simulink model "plant_block_2024"  (R2024b)
settings: Solver=ode1  StartTime=0.0  StopTime=3000  RelTol=1e-3  EnableMultiTasking=on
libraries: slpidlib x3
settings Model: SimulationMode=external  Creator=Dro  LastModifiedBy=s4580656
settings SolverCC: AlgebraicLoopSolver=TrustRegion
settings DataIOCC: LimitDataPoints=on  SaveFormat=Array  SignalLoggingSaveFormat=ModelDataLogs  ReturnWorkspaceOutputs=off  SignalLoggingName=sigsOut
settings OptimizationCC: ExpressionDepthLimit=2147483647  InitFltsAndDblsToZero=on
settings DebuggingCC: SaveWithParameterizedLinksMsg=none  UnderspecifiedInitializationDetection=Classic  MergeDetectMultiDrivingBlocksExec=none  SignalResolutionControl=TryResolveAllWithWarning  MultiTaskDSMMsg=warning  MultiTaskCondExecSysMsg=none  FcnCallInpInsideContextMsg=warning  UnconnectedInputMsg=warning  UnconnectedOutputMsg=warning  UnconnectedLineMsg=warning  StateNameClashWarn=warning  SFUnexpectedBacktrackingDiag=warning  SFNoUnconditionalDefaultTransitionDiag=warning  SFExecutionAtInitializationDiag=none  ArithmeticOperatorsInVariantConditions=warning
settings HardwareCC: ProdBitPerLong=64  ProdHWDeviceType=Intel->x86-64 (Linux 64)  TargetBitPerLong=64  TargetBitPerPointer=64  TargetIntDivRoundTo=Zero  TargetEndianess=LittleEndian  TargetWordSize=64  TargetHWDeviceType=Intel->x86-64
settings ModelReferenceCC: EnableRefExpFcnMdlSchedulingChecks=on  PropagateSignalLabelsOutOfModel=off
settings SFSimCC: SimUseLocalCustomCode=off  CustomCodeUndefinedFunction=UseInterfaceOnly
settings RTWCC: Description=Simulink Desktop Real-Time  SystemTargetFile=sldrt.tlc  TemplateMakefile=sldrt.tmf  RTWUseLocalCustomCode=off  RTWCompilerOptimization=on  GPUComputeCapability=3.5
settings CodeAppCC: MaxIdLength=95  StateflowObjectComments=on
settings SimulinkDesktopRealTimeCC: TargetLibSuffix=_sldrt.a  TargetPreCompLibLocation=C:\Program Files\MATLAB\R2024b\toolbox\sldrt\lib\win64  TargetLangStandard=C89/C90 (ANSI)  ModelReferenceCompliant=off  ParMdlRefBuildCompliant=on  CompOptLevelCompliant=off  SupportVariableSizeSignals=off
settings ConfigComp: CovMetricSettings=dw  CovSaveCumulativeToWorkspaceVar=on  CovSaveSingleToWorkspaceVar=on  CovExternalEMLEnable=off

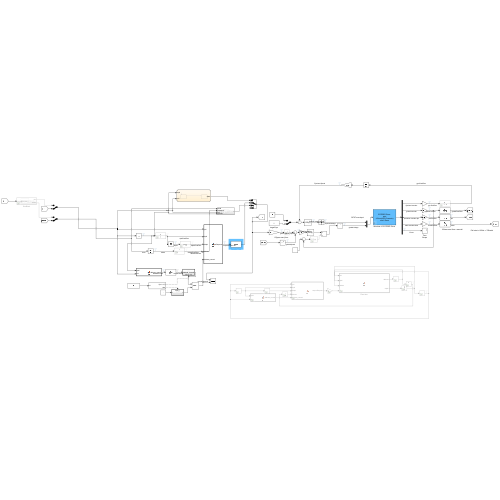
[thumbnail: Simulink's stored preview of the top-level diagram]
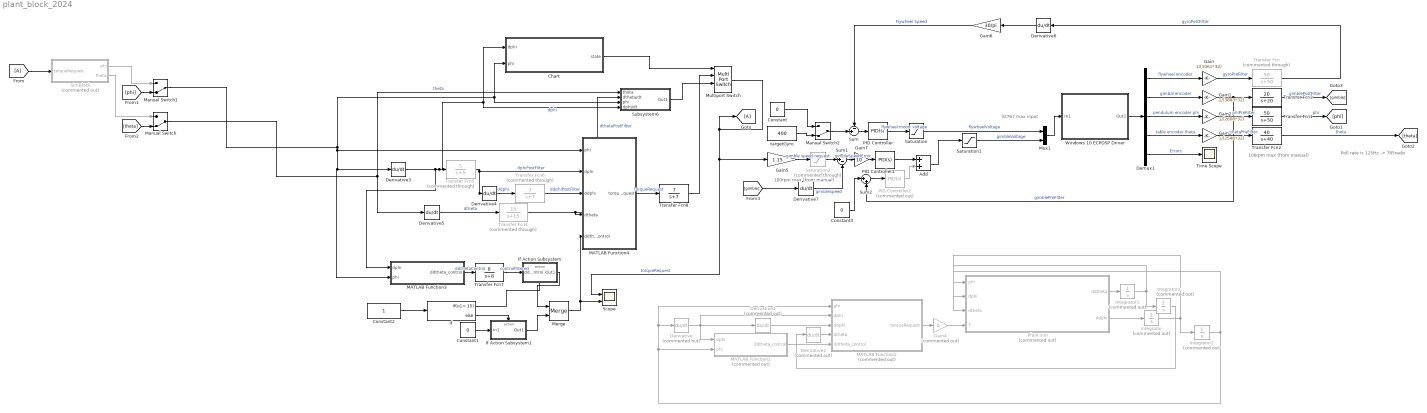
== system plant_block_2024 ==
  note: 100rpm max (from manual)
  note: 32767 max input
  note: Poll rate is 125Hz -> 785rad/s
  note: 100rpm max (from manual)
  Add : Sum
  Chart : Stateflow chart  TreatAsAtomicUnit=on
  Constant : Constant  Value=0
  Constant1 : Constant  Value=0
  Constant2 : Constant
  Constant3 : Constant  Value=0
  Demux1 : Demux  Outputs=5
      settings: DisplayOption=none
  Derivative : Derivative  Commented=on
  Derivative1 : Derivative  Commented=on
  Derivative2 : Derivative  Commented=on
  Derivative{3..7} (5 alike) : Derivative
  From : From
  Gain : Gain  Gain=1/(1061*32)
  Gain1 : Gain  Gain=1/(3883*32)
  Gain2 : Gain  Gain=1/(2608*32)
  Gain3 : Gain  Gain=1/(2546*32)
  Gain4 : Gain  Commented=on  Gain=0
  Gain5 : Gain  Gain=1.15
  Gain6 : Gain  Gain=30/pi
  Gain7 : Gain  Gain=10
  Goto : Goto
  If : If  IfExpression=u1< 15
  If Action Subsystem : Subsystem  TreatAsAtomicUnit=on
  If Action Subsystem1 : Subsystem  TreatAsAtomicUnit=on
  Integrator : Integrator  Commented=on
  Integrator1 : Integrator  Commented=on
  Integrator2 : Integrator  Commented=on  InitialCondition=pi
  Integrator3 : Integrator  Commented=on
  MATLAB Function1 : MATLAB Function  Commented=on  TreatAsAtomicUnit=on
  MATLAB Function2 : MATLAB Function  Commented=on  TreatAsAtomicUnit=on
  MATLAB Function3 : MATLAB Function  TreatAsAtomicUnit=on
  MATLAB Function4 : MATLAB Function  TreatAsAtomicUnit=on
  Manual Switch : ManualSwitch  CurrentSetting=0
  Manual Switch1 : ManualSwitch  CurrentSetting=0
  Manual Switch2 : ManualSwitch  CurrentSetting=0
  Merge : Merge  InitialOutput=[1]
  Multiport Switch : MultiPortSwitch  SaturateOnIntegerOverflow=off  InputSameDT=off
  Mux1 : Mux  Inputs=2
  PID Controller : slpidlib/PID Controller  Controller=PID  Form=Parallel  TimeDomain=Continuous-time  UseExternalTs=off  SampleTime=-1  IntegratorMethod=Forward Euler  FilterMethod=Forward Euler  ControllerParametersSource=internal  P=5500  I=100  UseKiTs=off  D=1  UseExternalDerivativeSource=off  N=100  UseFilter=on  TunerSelectOption=Transfer Function Based (PID Tuner App)  InitialConditionSource=internal  InitialConditionForIntegrator=0  InitialConditionForFilter=0  DifferentiatorICPrevScaledInput=0  ExternalReset=none  TrackingMode=off  Kt=1  LimitOutput=off  SatLimitsSource=internal  UpperSaturationLimit=32000  LowerSaturationLimit=-32000  LinearizeAsGain=on  AntiWindupMode=none  Kb=1  LimitIntegrator=off  UpperIntegratorSaturationLimit=inf  LowerIntegratorSaturationLimit=-inf  POutMin=[]  POutMax=[]  IOutMin=[]  IOutMax=[]  DOutMin=[]  DOutMax=[]  NOutMin=[]  NOutMax=[]  SumOutMin=[]  SumOutMax=[]  SaturationOutMin=[]  SaturationOutMax=[]  PParamMin=[]  PParamMax=[]  IParamMin=[]  IParamMax=[]  DParamMin=[]  DParamMax=[]  NParamMin=[]  NParamMax=[]  KbParamMin=[]  KbParamMax=[]  KtParamMin=[]  KtParamMax=[]  KbOutMin=[]  KbOutMax=[]  KtOutMin=[]  KtOutMax=[]  IntegratorOutMin=[]  IntegratorOutMax=[]  FilterOutMin=[]  FilterOutMax=[]  SumI1OutMin=[]  SumI1OutMax=[]  SumI2OutMin=[]  SumI2OutMax=[]  SumI3OutMin=[]  SumI3OutMax=[]  SumI4OutMin=[]  SumI4OutMax=[]  SumDOutMin=[]  SumDOutMax=[]  DifferentiatorOutMin=[]  DifferentiatorOutMax=[]  FilterDiffOutCoefMin=[]  FilterDiffOutCoefMax=[]  ReciprocalOutMin=[]  ReciprocalOutMax=[]  SumDenOutMin=[]  SumDenOutMax=[]  SumNumOutMin=[]  SumNumOutMax=[]  DivideOutMin=[]  DivideOutMax=[]  UdiffTsProdOutMin=[]  UdiffTsProdOutMax=[]  NTsProdOutMin=[]  NTsProdOutMax=[]  UintegralTsProdOutMin=[]  UintegralTsProdOutMax=[]  UngainTsProdOutMin=[]  UngainTsProdOutMax=[]  ClampingZeroOutDataTypeStr=Inherit: Inherit via back propagation  ClampingZeroOutMin=[]  ClampingZeroOutMax=[]  FilterDenConstantOutDataTypeStr=Inherit: Inherit via back propagation  FilterDenConstantOutMin=[]  FilterDenConstantOutMax=[]  PCopyOutDataTypeStr=Inherit: Inherit via back propagation  PCopyOutMin=[]  PCopyOutMax=[]  NCopyOutDataTypeStr=Inherit: Inherit via back propagation  NCopyOutMin=[]  NCopyOutMax=[]  IntegratorContinuousStateAttributes=''  IntegratorStateMustResolveToSignalObject=off  IntegratorRTWStateStorageClass=Auto  FilterContinuousStateAttributes=''  FilterStateMustResolveToSignalObject=off  FilterRTWStateStorageClass=Auto  ParallelPVariant=InternalParameters  IdealPVariant=Disabled  IVariant=InternalParameters  DVariant=InternalParameters  IntegratorVariant=Continuous  SatVariant=Disabled  AWVariant=Passthrough  PCopyVariant=Disabled  TRVariant=Disabled  FdbkBlocksVariant=Forward  IdealPFdbkVariant=Disabled  SatFdbkVariant=Disabled  DerivativeFilterVariant=ContFilter  NVariant=InternalParameters  NCopyVariant=Disabled  FilterICVariant=InternalICsFilter  IntegratorICVariant=InternalICs  ExternalResetVariant=Disabled  TRSumVariant=Passthrough  SumFdbkVariant=Disabled  SumVariant=Sum_PID  TsampFilterVariant=InternalTs  TsampNgainVariant=Passthrough  TsampIntegralVariant=Disabled_SignalSpec  ExternalSaturationOutDataTypeStr=Inherit: Same as second input  DerivativeSourceVariant=ErrorSignal  PreIntVariant=InternalPreInt
  PID Controller1 : slpidlib/PID Controller  Controller=PID  Form=Parallel  TimeDomain=Continuous-time  UseExternalTs=off  SampleTime=-1  IntegratorMethod=Forward Euler  FilterMethod=Forward Euler  ControllerParametersSource=internal  P=2500  I=50  UseKiTs=off  D=0  UseExternalDerivativeSource=off  N=100  UseFilter=on  TunerSelectOption=Transfer Function Based (PID Tuner App)  InitialConditionSource=internal  InitialConditionForIntegrator=0  InitialConditionForFilter=0  DifferentiatorICPrevScaledInput=0  ExternalReset=none  TrackingMode=off  Kt=1  LimitOutput=off  SatLimitsSource=internal  UpperSaturationLimit=23500  LowerSaturationLimit=-23500  LinearizeAsGain=on  AntiWindupMode=none  Kb=1  LimitIntegrator=off  UpperIntegratorSaturationLimit=inf  LowerIntegratorSaturationLimit=-inf  POutMin=[]  POutMax=[]  IOutMin=[]  IOutMax=[]  DOutMin=[]  DOutMax=[]  NOutMin=[]  NOutMax=[]  SumOutMin=[]  SumOutMax=[]  SaturationOutMin=[]  SaturationOutMax=[]  PParamMin=[]  PParamMax=[]  IParamMin=[]  IParamMax=[]  DParamMin=[]  DParamMax=[]  NParamMin=[]  NParamMax=[]  KbParamMin=[]  KbParamMax=[]  KtParamMin=[]  KtParamMax=[]  KbOutMin=[]  KbOutMax=[]  KtOutMin=[]  KtOutMax=[]  IntegratorOutMin=[]  IntegratorOutMax=[]  FilterOutMin=[]  FilterOutMax=[]  SumI1OutMin=[]  SumI1OutMax=[]  SumI2OutMin=[]  SumI2OutMax=[]  SumI3OutMin=[]  SumI3OutMax=[]  SumI4OutMin=[]  SumI4OutMax=[]  SumDOutMin=[]  SumDOutMax=[]  DifferentiatorOutMin=[]  DifferentiatorOutMax=[]  FilterDiffOutCoefMin=[]  FilterDiffOutCoefMax=[]  ReciprocalOutMin=[]  ReciprocalOutMax=[]  SumDenOutMin=[]  SumDenOutMax=[]  SumNumOutMin=[]  SumNumOutMax=[]  DivideOutMin=[]  DivideOutMax=[]  UdiffTsProdOutMin=[]  UdiffTsProdOutMax=[]  NTsProdOutMin=[]  NTsProdOutMax=[]  UintegralTsProdOutMin=[]  UintegralTsProdOutMax=[]  UngainTsProdOutMin=[]  UngainTsProdOutMax=[]  ClampingZeroOutDataTypeStr=Inherit: Inherit via back propagation  ClampingZeroOutMin=[]  ClampingZeroOutMax=[]  FilterDenConstantOutDataTypeStr=Inherit: Inherit via back propagation  FilterDenConstantOutMin=[]  FilterDenConstantOutMax=[]  PCopyOutDataTypeStr=Inherit: Inherit via back propagation  PCopyOutMin=[]  PCopyOutMax=[]  NCopyOutDataTypeStr=Inherit: Inherit via back propagation  NCopyOutMin=[]  NCopyOutMax=[]  IntegratorContinuousStateAttributes=''  IntegratorStateMustResolveToSignalObject=off  IntegratorRTWStateStorageClass=Auto  FilterContinuousStateAttributes=''  FilterStateMustResolveToSignalObject=off  FilterRTWStateStorageClass=Auto  ParallelPVariant=InternalParameters  IdealPVariant=Disabled  IVariant=InternalParameters  DVariant=InternalParameters  IntegratorVariant=Continuous  SatVariant=Disabled  AWVariant=Passthrough  PCopyVariant=Disabled  TRVariant=Disabled  FdbkBlocksVariant=Forward  IdealPFdbkVariant=Disabled  SatFdbkVariant=Disabled  DerivativeFilterVariant=ContFilter  NVariant=InternalParameters  NCopyVariant=Disabled  FilterICVariant=InternalICsFilter  IntegratorICVariant=InternalICs  ExternalResetVariant=Disabled  TRSumVariant=Passthrough  SumFdbkVariant=Disabled  SumVariant=Sum_PID  TsampFilterVariant=InternalTs  TsampNgainVariant=Passthrough  TsampIntegralVariant=Disabled_SignalSpec  ExternalSaturationOutDataTypeStr=Inherit: Same as second input  DerivativeSourceVariant=ErrorSignal  PreIntVariant=InternalPreInt
  PID Controller2 : slpidlib/PID Controller  Commented=on  Controller=PID  Form=Parallel  TimeDomain=Continuous-time  UseExternalTs=off  SampleTime=-1  IntegratorMethod=Forward Euler  FilterMethod=Forward Euler  ControllerParametersSource=internal  P=0  I=0  UseKiTs=off  D=0  UseExternalDerivativeSource=off  N=100  UseFilter=on  TunerSelectOption=Transfer Function Based (PID Tuner App)  InitialConditionSource=internal  InitialConditionForIntegrator=0  InitialConditionForFilter=0  DifferentiatorICPrevScaledInput=0  ExternalReset=none  TrackingMode=off  Kt=1  LimitOutput=off  SatLimitsSource=internal  UpperSaturationLimit=inf  LowerSaturationLimit=-inf  LinearizeAsGain=on  AntiWindupMode=none  Kb=1  LimitIntegrator=off  UpperIntegratorSaturationLimit=inf  LowerIntegratorSaturationLimit=-inf  POutMin=[]  POutMax=[]  IOutMin=[]  IOutMax=[]  DOutMin=[]  DOutMax=[]  NOutMin=[]  NOutMax=[]  SumOutMin=[]  SumOutMax=[]  SaturationOutMin=[]  SaturationOutMax=[]  PParamMin=[]  PParamMax=[]  IParamMin=[]  IParamMax=[]  DParamMin=[]  DParamMax=[]  NParamMin=[]  NParamMax=[]  KbParamMin=[]  KbParamMax=[]  KtParamMin=[]  KtParamMax=[]  KbOutMin=[]  KbOutMax=[]  KtOutMin=[]  KtOutMax=[]  IntegratorOutMin=[]  IntegratorOutMax=[]  FilterOutMin=[]  FilterOutMax=[]  SumI1OutMin=[]  SumI1OutMax=[]  SumI2OutMin=[]  SumI2OutMax=[]  SumI3OutMin=[]  SumI3OutMax=[]  SumI4OutMin=[]  SumI4OutMax=[]  SumDOutMin=[]  SumDOutMax=[]  DifferentiatorOutMin=[]  DifferentiatorOutMax=[]  FilterDiffOutCoefMin=[]  FilterDiffOutCoefMax=[]  ReciprocalOutMin=[]  ReciprocalOutMax=[]  SumDenOutMin=[]  SumDenOutMax=[]  SumNumOutMin=[]  SumNumOutMax=[]  DivideOutMin=[]  DivideOutMax=[]  UdiffTsProdOutMin=[]  UdiffTsProdOutMax=[]  NTsProdOutMin=[]  NTsProdOutMax=[]  UintegralTsProdOutMin=[]  UintegralTsProdOutMax=[]  UngainTsProdOutMin=[]  UngainTsProdOutMax=[]  ClampingZeroOutDataTypeStr=Inherit: Inherit via back propagation  ClampingZeroOutMin=[]  ClampingZeroOutMax=[]  FilterDenConstantOutDataTypeStr=Inherit: Inherit via back propagation  FilterDenConstantOutMin=[]  FilterDenConstantOutMax=[]  PCopyOutDataTypeStr=Inherit: Inherit via back propagation  PCopyOutMin=[]  PCopyOutMax=[]  NCopyOutDataTypeStr=Inherit: Inherit via back propagation  NCopyOutMin=[]  NCopyOutMax=[]  IntegratorContinuousStateAttributes=''  IntegratorStateMustResolveToSignalObject=off  IntegratorRTWStateStorageClass=Auto  FilterContinuousStateAttributes=''  FilterStateMustResolveToSignalObject=off  FilterRTWStateStorageClass=Auto  ParallelPVariant=InternalParameters  IdealPVariant=Disabled  IVariant=InternalParameters  DVariant=InternalParameters  IntegratorVariant=Continuous  SatVariant=Disabled  AWVariant=Passthrough  PCopyVariant=Disabled  TRVariant=Disabled  FdbkBlocksVariant=Forward  IdealPFdbkVariant=Disabled  SatFdbkVariant=Disabled  DerivativeFilterVariant=ContFilter  NVariant=InternalParameters  NCopyVariant=Disabled  FilterICVariant=InternalICsFilter  IntegratorICVariant=InternalICs  ExternalResetVariant=Disabled  TRSumVariant=Passthrough  SumFdbkVariant=Disabled  SumVariant=Sum_PID  TsampFilterVariant=InternalTs  TsampNgainVariant=Passthrough  TsampIntegralVariant=Disabled_SignalSpec  ExternalSaturationOutDataTypeStr=Inherit: Same as second input  DerivativeSourceVariant=ErrorSignal  PreIntVariant=InternalPreInt
  Plant sim : MATLAB Function  Commented=on  TreatAsAtomicUnit=on
  Saturation : Saturate  UpperLimit=30000  LowerLimit=-30000
  Saturation1 : Saturate  UpperLimit=30000  LowerLimit=-30000
  Saturation2 : Saturate  Commented=through  UpperLimit=15  LowerLimit=-15
  Scope : Scope  NumInputPorts=2
  SimBlock : Subsystem  Commented=on
  Subsystem6 : Subsystem
  Sum : Sum  Inputs=-+|
  Sum1 : Sum  Inputs=|+-
  Sum2 : Sum  Inputs=|++
  Time Scope : Scope
  Transfer Fcn : TransferFcn  Commented=through  Numerator=[50]  Denominator=[1 50]
  Transfer Fcn1 : TransferFcn  Numerator=[50]  Denominator=[1 50]
  Transfer Fcn2 : TransferFcn  Numerator=[40]  Denominator=[1 40]
  Transfer Fcn3 : TransferFcn  Numerator=[20]  Denominator=[1 20]
  Transfer Fcn4 : TransferFcn  Commented=through  Numerator=[15]  Denominator=[1 15]
  Transfer Fcn5 : TransferFcn  Commented=through  Numerator=[5]  Denominator=[1 5]
  Transfer Fcn6 : TransferFcn  Commented=through  Numerator=[7]  Denominator=[1 7]
  Transfer Fcn7 : TransferFcn  Numerator=[8]  Denominator=[1 8]
  Transfer Fcn8 : TransferFcn  Numerator=[7]  Denominator=[1 7]
  Windows 10 ECPDSP Driver : Subsystem  mask{BaseAddr='0x3F00', STime=0.008, TimeOutPer=500, HWAccess=on}
      mask prompts: BaseAddr "Base I/O Address"; STime "Sample Time (Sec)"; TimeOutPer "Timeout Period (500 ~ 2000)"; HWAccess "Hardware Access"
      mask Display: color('black');disp('ECPDSP Driver\n upto\n 4 Encs(ADC Channels)\n and 2 Dacs')
  targetGyro : Constant  Value=400
  wires:
  Mux1/1 -> Windows 10 ECPDSP Driver/1(In1)
  PID Controller/1 -> Saturation/1  "flywheel motor voltage"
  Demux1/1 -> Gain/1  "flywheel encoder"
  Demux1/2 -> Gain1/1  "gimbal encoder"
  Demux1/3 -> Gain2/1  "pendulum encoder phi"
  Demux1/4 -> Gain3/1  "table encoder theta"
  Sum1/1 -> Gain7/1  "gimbleSpeedError"
  Windows 10 ECPDSP Driver/1(Out1) -> Demux1/1
  Plant sim/2(ddphi) -> Integrator/1
  Plant sim/1(ddtheta) -> Integrator1/1
  Integrator/1 -> Plant sim/2(dphi), Integrator2/1
  Integrator1/1 -> Integrator3/1, Plant sim/3(dtheta)
  Integrator2/1 -> Plant sim/1(phi), MATLAB Function2/1(phi), Derivative/1, MATLAB Function1/2(phi)
  Derivative/1 -> Derivative1/1, MATLAB Function2/2(dphi), MATLAB Function1/1(dphi)
  MATLAB Function1/1(ddtheta_control) -> MATLAB Function2/5(ddtheta_control)
  Derivative1/1 -> MATLAB Function2/3(ddphi)
  Derivative2/1 -> MATLAB Function2/4(dtheta)
  Integrator3/1 -> Derivative2/1
  MATLAB Function2/1(torqueRequest) -> Gain4/1
  Gain4/1 -> Plant sim/4(T)
  MATLAB Function3/1(ddtheta_control) -> Transfer Fcn7/1  "ddthetaControl"
  Derivative5/1 -> Transfer Fcn4/1  "dtheta"
  Derivative4/1 -> Transfer Fcn6/1  "ddphi"
  Derivative3/1 -> MATLAB Function3/1(dphi), Subsystem6/4(dphi/dt), Chart/1(dphi), Transfer Fcn5/1  "dphi"
  Transfer Fcn2/1 -> [theta]  "theta"
  Gain2/1 -> Transfer Fcn1/1  "phiPreFilter"
  Sum/1 -> PID Controller/1
  targetGyro/1 -> Manual Switch2/2
  Gain/1 -> Transfer Fcn/1  "gyroPreFilter"
  Derivative6/1 -> Gain6/1
  Gain6/1 -> Sum/1  "Flywheel Speed"
  Gain5/1 -> Saturation2/1  "gimble speed request"
  Gain1/1 -> Transfer Fcn3/1, Sum2/2  "gimblePreFilter"
  Add/1 -> Saturation1/1
  Derivative7/1 -> Sum1/2  "gimbleSpeed"
  Saturation1/1 -> Mux1/2  "gimbleVoltage"
  Saturation2/1 -> Sum1/1
  Transfer Fcn1/1 -> [phi]  "phi"
  Manual Switch/1 -> Subsystem6/1(theta), Derivative5/1  "theta"
  Multiport Switch/1 -> Goto/1, Scope/1, Gain5/1  "torqueRequest"
  Manual Switch1/1 -> MATLAB Function4/1(phi), MATLAB Function3/2(phi), Derivative3/1, Subsystem6/3(phi), Chart/2(phi)
  Transfer Fcn3/1 -> [gimble]  "gimblePostFilter"
  Demux1/5 -> Time Scope/1  "Errors"
  Transfer Fcn/1 -> Derivative6/1  "gyroPostFilter"
  Gain3/1 -> Transfer Fcn2/1  "thetaPreFilter"
  SimBlock/1(phi) -> Manual Switch1/1
  SimBlock/2(theta) -> Manual Switch/1
  From/1 -> SimBlock/1(torqueRequest)
  [phi] -> Manual Switch1/2
  [gimble] -> Derivative7/1
  [theta] -> Manual Switch/2
  Merge/1 -> MATLAB Function4/5(ddtheta_control), Scope/2
  If Action Subsystem/1(Out1) -> Merge/1
  If/2 -> If Action Subsystem1/Action
  If/1 -> If Action Subsystem/Action
  Constant1/1 -> If Action Subsystem1/1(In1)
  If Action Subsystem1/1(Out1) -> Merge/2
  Constant2/1 -> If/1
  Transfer Fcn4/1 -> Subsystem6/2(dtheta/dt), MATLAB Function4/4(dtheta)  "dthetaPostFilter"
  Manual Switch2/1 -> Sum/2
  Constant/1 -> Manual Switch2/1
  Sum2/1 -> PID Controller2/1
  Constant3/1 -> Sum2/1
  PID Controller1/1 -> Add/1
  PID Controller2/1 -> Add/2
  Chart/1(state) -> Multiport Switch/1
  MATLAB Function4/1(torqueRequest) -> Transfer Fcn8/1  "torqueRequest"
  Subsystem6/1(Out1) -> Multiport Switch/3
  Transfer Fcn5/1 -> MATLAB Function4/2(dphi), Derivative4/1  "dphiPostFilter"
  Transfer Fcn6/1 -> MATLAB Function4/3(ddphi)  "ddphiPostFilter"
  Saturation/1 -> Mux1/1  "flywheelVoltage"
  Transfer Fcn7/1 -> If Action Subsystem/1(ddtheta_control)  "controlFiltered"
  Gain7/1 -> PID Controller1/1
  Transfer Fcn8/1 -> Multiport Switch/2

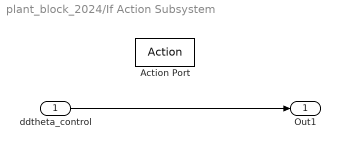
== system plant_block_2024/If Action Subsystem ==
  ddtheta_control : Inport
  Action Port : ActionPort  ActionPortLabel=if(u1< 15)
  Out1 : Outport
  wires:
  ddtheta_control/1 -> Out1/1

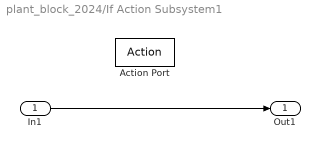
== system plant_block_2024/If Action Subsystem1 ==
  In1 : Inport
  Action Port : ActionPort  ActionPortLabel=else
  Out1 : Outport
  wires:
  In1/1 -> Out1/1

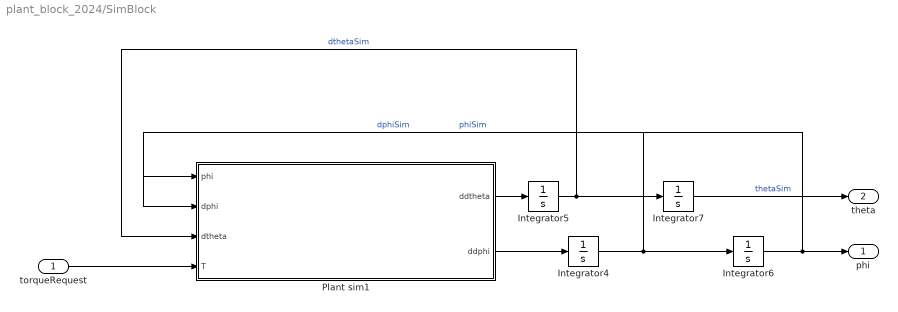
== system plant_block_2024/SimBlock ==
  torqueRequest : Inport
  Integrator4 : Integrator  InitialCondition=0.6  LimitOutput=on  UpperSaturationLimit=100  LowerSaturationLimit=-100
  Integrator5 : Integrator  InitialCondition=0.01  LimitOutput=on  UpperSaturationLimit=100  LowerSaturationLimit=-100
  Integrator6 : Integrator  InitialCondition=0.8*pi
  Integrator7 : Integrator  InitialCondition=0.01
  Plant sim1 : MATLAB Function  TreatAsAtomicUnit=on
  phi : Outport
  theta : Outport  Port=2
  wires:
  Integrator5/1 -> Integrator7/1, Plant sim1/3(dtheta)  "dthetaSim"
  Plant sim1/1(ddtheta) -> Integrator5/1
  Plant sim1/2(ddphi) -> Integrator4/1
  Integrator4/1 -> Plant sim1/2(dphi), Integrator6/1  "dphiSim"
  Integrator6/1 -> phi/1, Plant sim1/1(phi)  "phiSim"
  Integrator7/1 -> theta/1  "thetaSim"
  torqueRequest/1 -> Plant sim1/4(T)

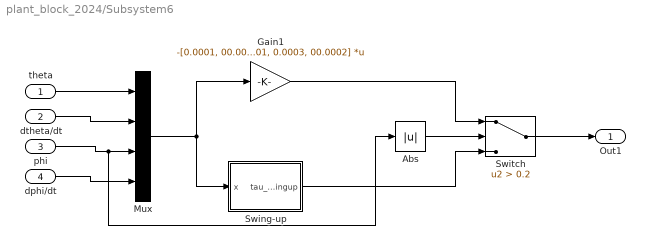
== system plant_block_2024/Subsystem6 ==
  theta : Inport
  dtheta/dt : Inport  Port=2
  phi : Inport  Port=3
  dphi/dt : Inport  Port=4
  Abs : Abs  SaturateOnIntegerOverflow=off
  Gain1 : Gain  Gain=-[0.0001, 00.0001, 0.0003, 00.0002]  Multiplication=Matrix(K*u)
  Mux : Mux
  Swing-up : MATLAB Function  TreatAsAtomicUnit=on
  Switch : Switch  Criteria=u2 > Threshold  Threshold=0.2  SaturateOnIntegerOverflow=off  InputSameDT=off
  Out1 : Outport
  wires:
  theta/1 -> Mux/1
  Mux/1 -> Gain1/1, Swing-up/1(x)
  dtheta/dt/1 -> Mux/2
  phi/1 -> Abs/1, Mux/3
  dphi/dt/1 -> Mux/4
  Abs/1 -> Switch/2
  Swing-up/1(tau_swingup) -> Switch/3
  Switch/1 -> Out1/1
  Gain1/1 -> Switch/1

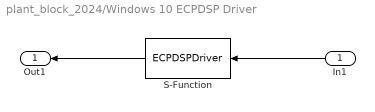
== system plant_block_2024/Windows 10 ECPDSP Driver ==
  In1 : Inport
  S-Function : S-Function  FunctionName=ECPDSPDriver  Parameters=BaseAddr,STime,TimeOutPer,HWAccess  SFunctionDeploymentMode=off  EnableBusSupport=off
  Out1 : Outport
  wires:
  In1/1 -> S-Function/1
  S-Function/1 -> Out1/1

== matlab function plant_block_2024/MATLAB Function1 ==
  data: dphi input; phi input; ddtheta_control output
function ddtheta_control = fcn(dphi, phi)
R = Rh
l = lcg;
r = 0; %reduced into J1_bar
M = 0; %reduced into J1_bar
g = grav;
c1 = 1; %friction of base
c2 = 0; %friction of pivot

J =  J1_bar% J - inertia of the table
Iyy = Jy 
I = Jz_bar%  I - inertia of the pendulum

k = 1
E = 0.5*I*dphi^2+m*g*l*(cos(phi)-1);
ddtheta_control = -k*E*dphi*cos(phi)/R;

== matlab function plant_block_2024/Plant sim ==
  data: phi input; ddtheta output; dphi input; dtheta input; T input; ddphi output
function [ddtheta, ddphi] = fcn(phi, dphi, dtheta, T)

R = Rh
l = lcg;
r = 0; %reduced into J1_bar
M = 0; %reduced into J1_bar
g = grav;
c1 = 1; %friction of base
c2 = 0; %friction of pivot

J =  J1_bar% J - inertia of the table
Iyy = Jy 
I = Jz_bar%  I - inertia of the pendulum

ddtheta = -(R*m*sin(phi)*dphi^2*l + dtheta*m*sin(2*phi)*dphi*l^2 + Iyy*dtheta*sin(2*phi)*dphi - R*ddphi*m*cos(phi)*l - T + c1*dtheta)/(m*R^2 - m*l^2*cos(phi)^2 + m*l^2 - Iyy*cos(phi)^2 + Iyy + J);
ddphi = -(c2*dphi - 0.5000*Iyy*dtheta^2*sin(2*phi) + g*l*m*sin(phi) - 0.5000*dtheta^2*l^2*m*sin(2*phi) + (R*l*m*cos(phi)*(R*m*sin(phi)*dphi^2*l + dtheta*m*sin(2*phi)*dphi*l^2 + Iyy*dtheta*sin(2*phi)*dphi - T + c1*dtheta))/(m*R^2 - m*l^2*cos(phi)^2 + m*l^2 - Iyy*cos(phi)^2 + Iyy + J))/(I + l^2*m - (R^2*l^2*m^2*cos(phi)^2)/(m*R^2 - m*l^2*cos(phi)^2 + m*l^2 - Iyy*cos(phi)^2 + Iyy + J))
y = u;

== matlab function plant_block_2024/MATLAB Function2 ==
  data: phi input; dphi input; ddphi input; dtheta input; torqueRequest output; ddtheta_control input
function torqueRequest = fcn(phi, dphi, ddphi,dtheta, ddtheta_control)
R = Rh;
l = lcg;
r = 0; %reduced into J1_bar
M = 0; %reduced into J1_bar
g = grav;
c1 = 1; %friction of base
c2 = 0; %friction of pivot

J =  J1_bar% J - inertia of the table
Iyy = Jy 
I = Jz_bar%  I - inertia of the pendulum

 torqueRequest = Iyy*ddtheta_control + J*ddtheta_control + c1*dtheta + ddtheta_control*m*R^2 + ddtheta_control*m*l^2 - Iyy*ddtheta_control*cos(phi)^2 + Iyy*dtheta*sin(2*phi)*dphi - ddtheta_control*m*l^2*cos(phi)^2 + m*sin(phi)*R*dphi^2*l + dtheta*m*sin(2*phi)*dphi*l^2 - ddphi*m*R*l*cos(phi)

== matlab function plant_block_2024/MATLAB Function3 ==
  data: dphi input; phi input; ddtheta_control output
function ddtheta_control = fcn(dphi, phi)
R = 0.3700
l = 0.2698
r = 0; %reduced into J1_bar
M = 0; %reduced into J1_bar
g = 9.81;
c1 = 1; %friction of base
c2 = 0; %friction of pivot

J =  0.1530 % J1_bar J - inertia of the table
Iyy = 5.5625e-05 %Jy 
I = 0.0131%Jz_bar%  I - inertia of the pendulum
m =     0.1580


k = 15

E = 0.5*I*dphi^2+m*g*l*(cos(phi)-1);
ddtheta_control = -k*E*dphi*cos(phi)/R;

== matlab function plant_block_2024/MATLAB Function4 ==
  data: phi input; dphi input; ddphi input; dtheta input; torqueRequest output; ddtheta_control input
function torqueRequest = fcn(phi, dphi, ddphi,dtheta, ddtheta_control)
R = 0.3700
l = 0.2698
r = 0; %reduced into J1_bar
M = 0; %reduced into J1_bar
g = 9.81;
c1 = 1; %friction of base
c2 = 0; %friction of pivot

J =  0.1530 % J1_bar J - inertia of the table
Iyy = 5.5625e-05 %Jy 
I = 0.0131%Jz_bar%  I - inertia of the pendulum
m =     0.1580


torqueRequest = Iyy*ddtheta_control + J*ddtheta_control + c1*dtheta + ddtheta_control*m*R^2 + ddtheta_control*m*l^2 - Iyy*ddtheta_control*cos(phi)^2 + Iyy*dtheta*sin(2*phi)*dphi - ddtheta_control*m*l^2*cos(phi)^2 + m*sin(phi)*R*dphi^2*l + dtheta*m*sin(2*phi)*dphi*l^2 - ddphi*m*R*l*cos(phi)

== matlab function plant_block_2024/SimBlock/Plant sim1 ==
  data: phi input; ddtheta output; dphi input; dtheta input; T input; ddphi output
function [ddtheta, ddphi] = fcn(phi, dphi, dtheta, T)

R = 0.3700
l = 0.2698
r = 0; %reduced into J1_bar
M = 0; %reduced into J1_bar
g = 9.81;
c1 = 1; %friction of base
c2 = 0; %friction of pivot

J =  0.1530 % J1_bar J - inertia of the table
Iyy = 5.5625e-05 %Jy 
I = 0.0131%Jz_bar%  I - inertia of the pendulum
m =     0.1580
ddphi = -(c2*dphi - 0.5000*Iyy*dtheta^2*sin(2*phi) + g*l*m*sin(phi) - 0.5000*dtheta^2*l^2*m*sin(2*phi) + (R*l*m*cos(phi)*(R*m*sin(phi)*dphi^2*l + dtheta*m*sin(2*phi)*dphi*l^2 + Iyy*dtheta*sin(2*phi)*dphi - T + c1*dtheta))/(m*R^2 - m*l^2*cos(phi)^2 + m*l^2 - Iyy*cos(phi)^2 + Iyy + J))/(I + l^2*m - (R^2*l^2*m^2*cos(phi)^2)/(m*R^2 - m*l^2*cos(phi)^2 + m*l^2 - Iyy*cos(phi)^2 + Iyy + J))

ddtheta = -(R*m*sin(phi)*dphi^2*l + dtheta*m*sin(2*phi)*dphi*l^2 + Iyy*dtheta*sin(2*phi)*dphi - R*ddphi*m*cos(phi)*l - T + c1*dtheta)/(m*R^2 - m*l^2*cos(phi)^2 + m*l^2 - Iyy*cos(phi)^2 + Iyy + J);

== stateflow chart plant_block_2024/Chart ==
  state SwingUp
    state=1
  state Catch
    state=2
  (default) -> SwingUp
  SwingUp -> Catch : [mod(phi, 2*pi)<-abs(pi/18) && abs(dphi)<1]
  data: dphi input; phi input; state output

== matlab function plant_block_2024/Subsystem6/Swing-up ==
  data: x input; tau_swingup output
function tau_swingup = fcn(x)
%--------------------------------------------------------------------------
% Swing-up controller based on energy
%--------------------------------------------------------------------------
% Inputs:
%   x - State vector [cart position; cart velocity; pendulum angle (UP=0); pendulum angular velocity]
% Outputs:
%   tau_swingup - Control torque (or force) to apply
%--------------------------------------------------------------------------

% --- 1. Define Physical Constants ---
% NOTE: Replace these with the actual measured values for your system
M  = 0.127;     % Mass of the pendulum (kg)
lc = 0.15;      % Distance to pendulum's center of mass (m)
g  = 9.81;      % Gravity (m/s^2)

% --- 2. Define Controller Gain ---
% This is the main parameter to TUNE. Start with a small value
k = 1000;

% --- 3. Extract States from Input Vector ---
% Note: LQR uses phi = 0 as UP, but this controller uses phi = 0 as DOWN
phi_LQR = x(3);
dphi    = x(4);

% Convert angle so that phi = 0 corresponds to DOWN position
phi = phi_LQR + pi;

% --- 4. Calculate Energy ---
% Total energy of the pendulum (kinetic + potential)
E_current = 0.5 * M * (lc * dphi)^2 - M * g * lc * cos(phi);
E_target  = M * g * lc;  % Desired potential energy at the UP position
E_error   = E_current - E_target;

% --- 5. Apply the Control Law ---
% Calculate commanded acceleration (proportional to torque/force)
% Use sign(dphi * cos(phi)) for direction robustness
accel_cmd = k * E_error * sign(dphi * cos(phi));

% Optional: Add saturation to limit torque magnitude
max_accel = 20.0;  % Another tunable parameter
if abs(accel_cmd) > max_accel
    accel_cmd = sign(accel_cmd) * max_accel;
end

% --- Output Control Torque ---
tau_swingup = accel_cmd;

end
